simulink model "Controller_sim"  (R2021a)
settings: Solver=VariableStepAuto  StartTime=0.0  StopTime=30  RelTol=1e-3
values from neighbouring files (symbols this model uses):
  F_mimo = -place(A,B,Desired_poles)    [SS_MIMO.m]    (also in controller_code.m = [-1.4629         0         0         0   -2.7429         0  )
  L_mimo = -place(A',C',Desired_poles_obs)'    [SS_MIMO.m]
  sys_mimo = ss(A,B,C,0)    [SS_MIMO.m]
undefined symbols (not defined in the file or in its folder): Fa, Fg, M, N
libraries: simulink_extras x3
settings Model: Creator=krist  LastModifiedBy=mozzr
settings SolverCC: AlgebraicLoopSolver=TrustRegion
settings DebuggingCC: SFMachineParentedDataDiag=warning

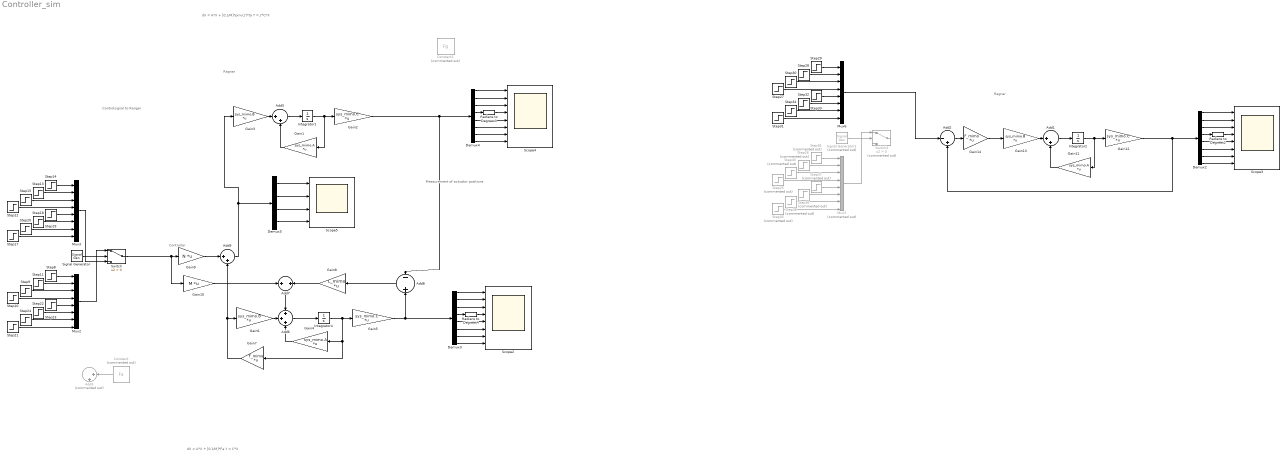
== system Controller_sim ==
  note: Ragnar
  note: Controller
  note: Measurement of
      | actuator positions
  note: Controlsignal
      | to Rangar
  note: dX = A*X + [0;1/M]*pinv(J')*ta
      | Y = J'*C*X
  note: dX = A*X + [0;1/M]*Fa
      | Y = C*X
  note: Ragnar
  Add1 : Sum  Inputs=|++
  Add2 : Sum  Inputs=|-+
  Add3 : Sum  Commented=on  Inputs=|++
  Add5 : Sum  Inputs=|++
  Add6 : Sum  Inputs=+++
  Add7 : Sum
  Add8 : Sum  Inputs=-+
  Add9 : Sum  Inputs=|++
  Constant : Constant  Commented=on  Value=Fa
  Constant1 : Constant  Commented=on  Value=Fg
  Demux2 : Demux  Outputs=8
  Demux3 : Demux  Outputs=8
  Demux4 : Demux  Outputs=8
  Demux5 : Demux
  Gain1 : Gain  Gain=sys_mimo.A  Multiplication=Matrix(K*u)
  Gain10 : Gain  Gain=M  Multiplication=Matrix(K*u)
  Gain11 : Gain  Gain=sys_mimo.A  Multiplication=Matrix(K*u)
  Gain12 : Gain  Gain=sys_mimo.C  Multiplication=Matrix(K*u)
  Gain13 : Gain  Gain=sys_mimo.B  Multiplication=Matrix(K*u)
  Gain14 : Gain  Gain=F_mimo  Multiplication=Matrix(K*u)
  Gain2 : Gain  Gain=sys_mimo.C  Multiplication=Matrix(K*u)
  Gain3 : Gain  Gain=sys_mimo.B  Multiplication=Matrix(K*u)
  Gain4 : Gain  Gain=sys_mimo.A  Multiplication=Matrix(K*u)
  Gain5 : Gain  Gain=sys_mimo.C  Multiplication=Matrix(K*u)
  Gain6 : Gain  Gain=sys_mimo.B  Multiplication=Matrix(K*u)
  Gain7 : Gain  Gain=F_mimo  Multiplication=Matrix(K*u)
  Gain8 : Gain  Gain=L_mimo  Multiplication=Matrix(K*u)
  Gain9 : Gain  Gain=N  Multiplication=Matrix(K*u)
  Integrator1 : Integrator  InitialCondition=[0 0.5 -0.4 deg2rad(90) 0 0 0 0]
  Integrator2 : Integrator  InitialCondition=[0 0.5 -0.4 deg2rad(90) 0 0 0 0]
  Integrator4 : Integrator  InitialCondition=[0 0.5 -0.4 deg2rad(90) 0 0 0 0]
  Mux2 : Mux  Inputs=8
  Mux3 : Mux  Inputs=8
  Mux5 : Mux  Commented=on  Inputs=8
  Mux6 : Mux  Inputs=8
  Radians to Degrees2 : simulink_extras/Transformations/Radians to Degrees
  Radians to Degrees3 : simulink_extras/Transformations/Radians to Degrees
  Radians to Degrees4 : simulink_extras/Transformations/Radians to Degrees
  Scope2 : Scope  NumInputPorts=8
  Scope3 : Scope  NumInputPorts=8
  Scope4 : Scope  NumInputPorts=8
  Scope5 : Scope  NumInputPorts=4
  Signal Generator : SignalGenerator  WaveForm=square  Frequency=0.4  Units=rad/sec
  Signal Generator2 : SignalGenerator  Commented=on  WaveForm=square  Frequency=0.4  Units=rad/sec
  Step10 : Step  Time=0  Before=deg2rad(85)  After=deg2rad(85)  SampleTime=1
  Step11 : Step  Time=0  Before=0.51  After=0.51  SampleTime=1
  Step12 : Step  Time=0  Before=deg2rad(90)  After=deg2rad(90)  SampleTime=1
  Step13 : Step  Time=0  Before=0.5  After=0.5  SampleTime=1
  Step{14,17..24,29,31..34} (14 alike) : Step  Time=0  After=0  SampleTime=1
  Step15 : Step  Time=0  Before=-0.4  After=-0.4  SampleTime=1
  Step25 : Step  Commented=on  Time=0  Before=deg2rad(85)  After=deg2rad(85)  SampleTime=1
  Step26 : Step  Commented=on  Time=0  Before=0.51  After=0.51  SampleTime=1
  Step27 : Step  Time=0  Before=deg2rad(90)  After=deg2rad(90)  SampleTime=1
  Step28 : Step  Time=0  Before=0.5  After=0.5  SampleTime=1
  Step30 : Step  Time=0  Before=-0.4  After=-0.4  SampleTime=1
  Step{35..38} (4 alike) : Step  Commented=on  Time=0  After=0  SampleTime=1
  Step39 : Step  Commented=on  Time=0  Before=0.01  After=0.01  SampleTime=1
  Step40 : Step  Commented=on  Time=0  Before=-0.41  After=-0.41  SampleTime=1
  Step8 : Step  Time=0  Before=0.01  After=0.01  SampleTime=1
  Step9 : Step  Time=0  Before=-0.41  After=-0.41  SampleTime=1
  Switch : Switch  Criteria=u2 > Threshold
  Switch2 : Switch  Commented=on  Criteria=u2 > Threshold
  wires:
  Add8/1 -> Gain8/1
  Gain8/1 -> Add7/2
  Gain10/1 -> Add7/1
  Gain1/1 -> Add5/2
  Integrator1/1 -> Gain1/1, Gain2/1
  Add5/1 -> Integrator1/1
  Gain3/1 -> Add5/1
  Gain9/1 -> Add9/1
  Add6/1 -> Integrator4/1
  Gain4/1 -> Add6/3
  Add7/1 -> Add6/1
  Gain6/1 -> Add6/2
  Integrator4/1 -> Gain4/1, Gain7/1, Gain5/1
  Signal Generator/1 -> Switch/2
  Step10/1 -> Mux2/4
  Step9/1 -> Mux2/3
  Step8/1 -> Mux2/1
  Step11/1 -> Mux2/2
  Step12/1 -> Mux3/4
  Step15/1 -> Mux3/3
  Step14/1 -> Mux3/1
  Step13/1 -> Mux3/2
  Mux2/1 -> Switch/1
  Mux3/1 -> Switch/3
  Switch/1 -> Gain10/1, Gain9/1
  Gain13/1 -> Add1/1
  Gain11/1 -> Add1/2
  Add1/1 -> Integrator2/1
  Integrator2/1 -> Gain11/1, Gain12/1
  Gain12/1 -> Add2/2, Demux2/1
  Demux2/4 -> Radians to Degrees2/1
  Demux2/3 -> Scope3/3
  Demux2/2 -> Scope3/2
  Demux2/1 -> Scope3/1
  Demux2/5 -> Scope3/5
  Demux2/6 -> Scope3/6
  Demux2/8 -> Scope3/8
  Demux4/8 -> Scope4/8
  Demux4/3 -> Scope4/3
  Demux4/2 -> Scope4/2
  Demux4/6 -> Scope4/6
  Demux4/5 -> Scope4/5
  Demux4/1 -> Scope4/1
  Demux4/7 -> Scope4/7
  Demux2/7 -> Scope3/7
  Radians to Degrees2/1 -> Scope3/4
  Demux4/4 -> Radians to Degrees3/1
  Radians to Degrees3/1 -> Scope4/4
  Step18/1 -> Mux3/6
  Step17/1 -> Mux3/8
  Step20/1 -> Mux3/7
  Step19/1 -> Mux3/5
  Step23/1 -> Mux2/5
  Step22/1 -> Mux2/6
  Step24/1 -> Mux2/7
  Step21/1 -> Mux2/8
  Constant/1 -> Add3/2
  Gain7/1 -> Gain6/1, Add9/2
  Demux5/4 -> Scope5/4
  Demux5/1 -> Scope5/1
  Demux5/3 -> Scope5/3
  Demux5/2 -> Scope5/2
  Demux3/1 -> Scope2/1
  Demux3/2 -> Scope2/2
  Demux3/3 -> Scope2/3
  Demux3/8 -> Scope2/8
  Demux3/6 -> Scope2/6
  Radians to Degrees4/1 -> Scope2/4
  Demux3/4 -> Radians to Degrees4/1
  Demux3/7 -> Scope2/7
  Demux3/5 -> Scope2/5
  Gain5/1 -> Demux3/1, Add8/2
  Add9/1 -> Demux5/1, Gain3/1
  Gain2/1 -> Demux4/1, Add8/1
  Add2/1 -> Gain14/1
  Gain14/1 -> Gain13/1
  Step28/1 -> Mux6/2
  Step26/1 -> Mux5/2
  Signal Generator2/1 -> Switch2/2
  Step27/1 -> Mux6/4
  Step34/1 -> Mux6/7
  Mux5/1 -> Switch2/1
  Step39/1 -> Mux5/1
  Step38/1 -> Mux5/7
  Step29/1 -> Mux6/1
  Step35/1 -> Mux5/8
  Step37/1 -> Mux5/5
  Step40/1 -> Mux5/3
  Step25/1 -> Mux5/4
  Step33/1 -> Mux6/5
  Step36/1 -> Mux5/6
  Step31/1 -> Mux6/8
  Step30/1 -> Mux6/3
  Step32/1 -> Mux6/6
  Mux6/1 -> Add2/1
